simulink model "MATLABfunction"  (R2022b)
settings: Solver=FixedStepAuto  StartTime=0.0  StopTime=10.0  RelTol=1e-3
undefined symbols (not defined in the file): h, km, m, s
libraries: simulink_extras x3, aerolibconvert2 x3, autolibshared x2, vehdynlibsteering x1, simulink x1
settings Model: Creator=Lenovo  LastModifiedBy=Lenovo
settings SolverCC: EnableFixedStepZeroCrossing=on

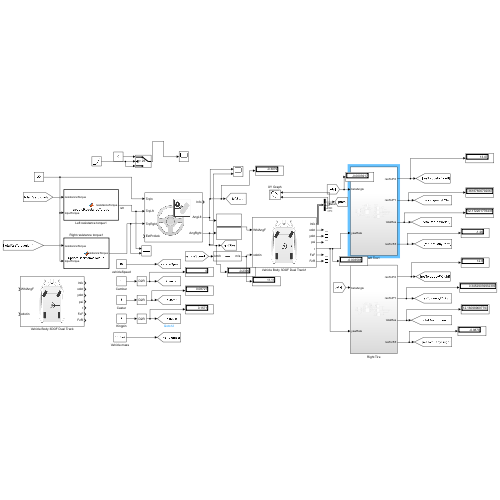
[thumbnail: Simulink's stored preview of the top-level diagram]
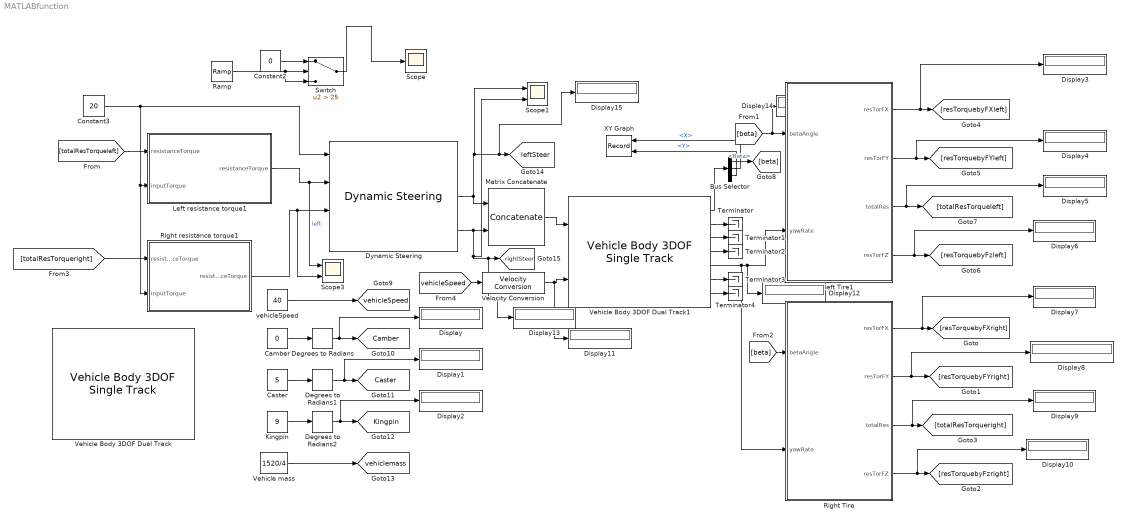
== system MATLABfunction ==
  Bus Selector : BusSelector  OutputSignals=BdyFrm.Geom.Ang.Beta,InertFrm.Cg.Disp.X,InertFrm.Cg.Disp.Y
  Camber : Constant  Value=0
  Caster : Constant  Value=5
  Constant2 : Constant  Value=0
  Constant3 : Constant  Value=20
  Degrees to Radians : simulink_extras/Transformations/Degrees to Radians
  Degrees to Radians1 : simulink_extras/Transformations/Degrees to Radians
  Degrees to Radians2 : simulink_extras/Transformations/Degrees to Radians
  Display{,1..15} (16 alike) : Display
  Dynamic Steering : vehdynlibsteering/Dynamic Steering  StrgType=Rack and pinion  StrgRatioType=Constant  PwrAst=off  Loc=Front  TrckWdth=1  WhlBase=1.524  StrgRng=1.25*pi  StrgAngBpts="[-6.2832   -5.0265   -3.7699   -2.5133   -1.2566         0    1.2566    2.5133    3.7699    5.0265    6.2832]"  StrgRatioTbl=|  StrgRatio=13.5  StrgArmLngth=0.1  RckCsLngth=0.5  TieRodLngth=0.248  D=0.2  PnnRadiusTbl="[0.0055    0.0055    0.0056    0.0057    0.0057    0.0057    0.0058    0.0057    0.0056    0.0055    0.0055]"  PnnRadius=0.0057  RodLngth=0.1  ParaArmLngth=0.9  J1=0.1  J2=0.01  beta_u=0.1  beta_l=0.1  b1=0.001  k1=30  b2=1  b3=0.001  theta_o=0  omega_o=0  FricTrq=0  TrqBpts=[-100 0 100]  VehSpdBpts=[0 20]  TrqTbl=[0 -100;0 0;0 100]  TrqLmt=100  PwrLmt=1000  Eta=1  omega_c=200  aMode=2
      | [13.5000   13.3750   13.2500   13.1250   13.0000   13.0000   13.0000   13.1250   13.2500   13.3750   13.5000
      | ]
  Kingpin : Constant  Value=9
  Left resistance torque1 : MATLAB Function  TreatAsAtomicUnit=on
  Matrix Concatenate : Concatenate  ConcatenateDimension=2
  Ramp : simulink/Sources/Ramp  slope=1  start=0  InitialOutput=5
  Right Tire : Subsystem
  Right resistance torque1 : MATLAB Function  TreatAsAtomicUnit=on
  Scope : Scope
  Scope1 : Scope  NumInputPorts=2
  Scope3 : Scope  NumInputPorts=2
  Switch : Switch  Criteria=u2 > Threshold  Threshold=25  SaturateOnIntegerOverflow=off  InputSameDT=off
  Terminator{,1..4} (5 alike) : Terminator
  Vehicle Body 3DOF Dual Track : autolibshared/Vehicle Body 3DOF Single Track  trackMode=Dual  inputMode=External longitudinal velocity  frontSteerMode=on  rearSteerMode=off  windMode=off  muMode=off  extFMode=off  extMMode=off  htchFMode=off  htchMMode=off  extXo=off  extpsio=off  extxdoto=off  extro=off  extYo=off  extTamb=off  extydoto=off  aMode=2  NF=2  NR=2  m=1520  a=1.4  b=1.6  h=0.35  dh=1  hh=0.2  X_o=0  xdot_o=0  CalphaMode=off  sigmaMode=on  d=0  hl=0  w=[1.4,1.4]  Cy_f=12e3  Cy_r=11e3  sigma_f=.1  sigma_r=.1  alpha_f_brk=[-.1 .1]  Cy_f_data=[-9e3 9e3]  alpha_r_brk=[-.1 .1]  Cy_r_data=[-9e3 9e3]  Y_o=0  ydot_o=0  Izz=4000  psi_o=0  r_o=0  Af=2  Cd=.3  Cl=.1  Cpm=.1  beta_w=[0 0.01:0.01:0.3]  Cs=[0:0.03:0.9]  Cym=[0 1e-6:0.01:0.3]  Pabs=101325  Tair=273  g=9.81  mu=1  xdot_tol=.01  Fznom=5000  Fxtire_sat=7e4  Fytire_sat=7e4  longOff=0  latOff=0  vertOff=0  wrapAng=off
      settings: LibrarySourceBlock=vehdynlibeom/Vehicle Body 3DOF Dual Track
  Vehicle Body 3DOF Dual Track1 : autolibshared/Vehicle Body 3DOF Single Track  trackMode=Dual  inputMode=External longitudinal velocity  frontSteerMode=on  rearSteerMode=off  windMode=off  muMode=off  extFMode=off  extMMode=off  htchFMode=off  htchMMode=off  extXo=off  extpsio=off  extxdoto=off  extro=off  extYo=off  extTamb=off  extydoto=off  aMode=2  NF=2  NR=2  m=1520  a=1.148  b=1.402  h=0.35  dh=1  hh=0.2  X_o=0  xdot_o=0  CalphaMode=off  sigmaMode=on  d=0  hl=0  w=[1.2,1.2]  Cy_f=350  Cy_r=12e3  sigma_f=.1  sigma_r=.1  alpha_f_brk=[-.1 .1]  Cy_f_data=[-9e3 9e3]  alpha_r_brk=[-.1 .1]  Cy_r_data=[-9e3 9e3]  Y_o=0  ydot_o=0  Izz=4000  psi_o=0  r_o=0  Af=2  Cd=.3  Cl=.1  Cpm=.1  beta_w=[0:0.01:0.3]  Cs=[0:0.03:0.9]  Cym=[0:0.01:0.3]  Pabs=101325  Tair=273  g=9.81  mu=1  xdot_tol=.01  Fznom=5000  Fxtire_sat=7e4  Fytire_sat=7e4  longOff=0  latOff=0  vertOff=0  wrapAng=off
  Vehicle mass : Constant  Value=1520/4
  Velocity Conversion : aerolibconvert2/Velocity Conversion  IU=km/h  OU=m/s
  XY Graph : Record  FileSettingsInternal="{\"entries\":[{\"content\":{\"excelSettings\":{\"content\":{},\"type\":\"Streamout.ExcelSettings\"}},\"type\":\"Streamout.FileSettingStorage\",\"uuid\":\"bec896f1-d56a-48de-90cf-f78405374d8f\"}],\"packageUris\":[\"http://schema.mathworks.com/mf0/streamout_blocks/R2020a\"],\"version\":\"1.0\"}"  Layout=[1 1]  SignalsInternal="{\"entries\":[{\"content\":{\"signals\":[{\"content\":{\"blockPath\":[\"untitled/XY Graph\"],\"channel\":[],\"dimensions\":[1],\"domain\":\"untitled/XY Graph\",\"lineColor\":\"#a2142f\",\"plots\":[1],\"port\":1,\"sid\":[\"\"],\"signalID\":30127,\"signalName\":\"<X>\"},\"type\":\"RecordBlkView.Signal\",\"uuid\":\"c8050bcf-ab5d-494c-af83-4e53599decc2\"},{\"content\":{\"blockPath\":[\"untitled/XY Graph\"],\"channel\":[],\"dimensions\":[1],\"domain\":\"untitled/XY Graph\",\"lineColor\":\"#139fff\",\"plots\":[1],\"port\":2,\"sid\":[\"\"],\"signalID\":30131,\"signalName\":\"<Y>\"},\"type\":\"RecordBlkView.Signal\",\"uuid\":\"10e66e42-d777-49f9-8d8c-30872f4fdeb7\"}]},\"type\":\"RecordBlkView.InputSignals\",\"uuid\":\"4fc47762-2255-40e3-9f9f-7b4ae2eb3bc2\"}],\"packageUris\":[\"http://schema.mathworks.com/mf0/streamout_blocks/R2020a\"],\"version\":\"1.0\"}"  VisualizationBindings="{\"xyplotplugin\":{\"info\":[{\"series\":[{\"bindingParametersList\":[{\"parameter\":\"X-Axis\",\"signalID\":30127,\"signalName\":\"<X>\"},{\"parameter\":\"Y-Axis\",\"signalID\":30131,\"signalName\":\"<Y>\"}],\"seriesID\":15033}],\"subplotID\":1}]}}"  CompatibilityTag=XY
  left Tire1 : Subsystem
  vehicleSpeed : Constant  Value=40
  tag scope: Camber=global, Caster=global, Kingpin=global, leftSteer=global, rightSteer=global, vehicleSpeed=global, vehiclemass=global
  wires:
  [beta] -> Right Tire/1(betaAngle)
  Dynamic Steering/2 -> Matrix Concatenate/1, Scope1/1, Display15/1, [leftSteer]
  Dynamic Steering/3 -> Scope1/2, [rightSteer], Display13/1, Matrix Concatenate/2
  Matrix Concatenate/1 -> Vehicle Body 3DOF Dual Track1/1
  Right Tire/1(resTorFX) -> Display7/1, [resTorquebyFXright]
  Right Tire/2(resTorFY) -> Display8/1, [resTorquebyFYright]
  Right Tire/4(resTorFZ) -> Display10/1, [resTorquebyFzright]
  Right Tire/3(totalRes) -> Display9/1, [totalResTorqueright]
  Vehicle Body 3DOF Dual Track1/5 -> Display12/1, left Tire1/2(yawRate), Right Tire/2(yawRate)
  Vehicle Body 3DOF Dual Track1/1 -> Bus Selector/1
  Bus Selector/1 -> [beta]  "<Beta>"
  [beta] -> Display14/1, left Tire1/1(betaAngle)
  Vehicle Body 3DOF Dual Track1/2 -> Terminator/1
  Vehicle Body 3DOF Dual Track1/3 -> Terminator1/1
  Vehicle Body 3DOF Dual Track1/4 -> Terminator2/1
  Vehicle Body 3DOF Dual Track1/6 -> Terminator3/1
  Vehicle Body 3DOF Dual Track1/7 -> Terminator4/1
  vehicleSpeed/1 -> [vehicleSpeed]
  Camber/1 -> Degrees to Radians/1
  Caster/1 -> Degrees to Radians1/1
  Kingpin/1 -> Degrees to Radians2/1
  Vehicle mass/1 -> [vehiclemass]
  Degrees to Radians/1 -> Display/1, [Camber]
  Degrees to Radians1/1 -> Display1/1, [Caster]
  Degrees to Radians2/1 -> Display2/1, [Kingpin]
  [vehicleSpeed] -> Velocity Conversion/1
  Velocity Conversion/1 -> Display11/1, Vehicle Body 3DOF Dual Track1/2
  Constant2/1 -> Switch/1
  Ramp/1 -> Switch/3, Switch/2
  Switch/1 -> Scope/1
  Bus Selector/2 -> XY Graph/1  "<X>"
  Bus Selector/3 -> XY Graph/2  "<Y>"
  left Tire1/3(totalRes) -> Display5/1, [totalResTorqueleft]
  left Tire1/4(resTorFZ) -> Display6/1, [resTorquebyFzleft]
  left Tire1/2(resTorFY) -> Display4/1, [resTorquebyFYleft]
  left Tire1/1(resTorFX) -> Display3/1, [resTorquebyFXleft]
  [totalResTorqueleft] -> Left resistance torque1/1("resistanceTorque ")
  Constant3/1 -> Right resistance torque1/2(inputTorque), Left resistance torque1/2(inputTorque), Dynamic Steering/1
  Left resistance torque1/1(resistanceTorque) -> Scope3/1, Dynamic Steering/2  "left"
  [totalResTorqueright] -> Right resistance torque1/1("resistanceTorque ")
  Right resistance torque1/1(resistanceTorque) -> Scope3/2, Dynamic Steering/3

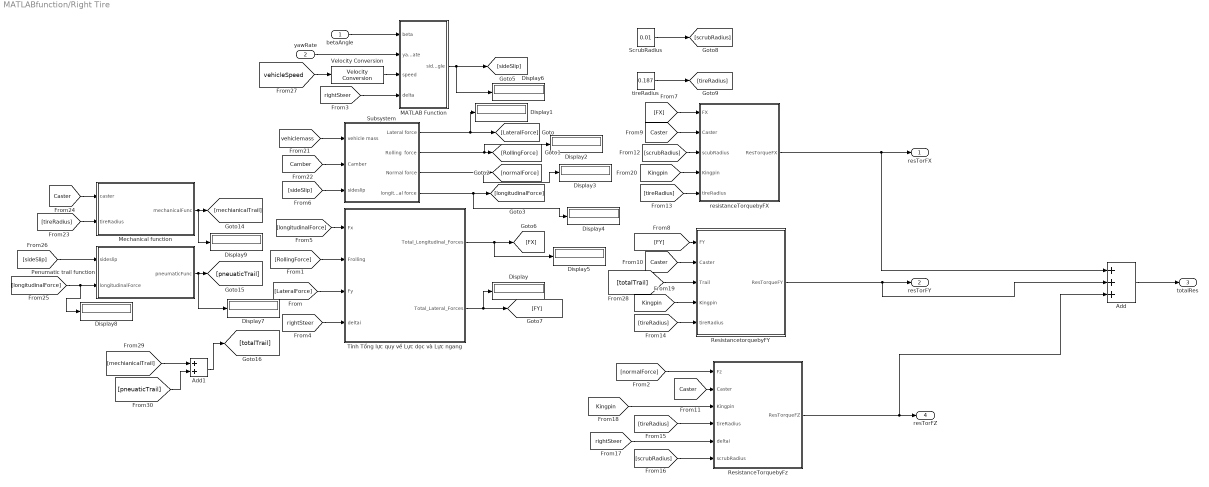
== system MATLABfunction/Right Tire ==
  betaAngle : Inport
  yawRate : Inport  Port=2
  Add : Sum  Inputs=+++
  Add1 : Sum
  Display{,1..9} (10 alike) : Display
  MATLAB Function : MATLAB Function  TreatAsAtomicUnit=on
  Mechanical function : MATLAB Function  TreatAsAtomicUnit=on
  Penumatic trail function : MATLAB Function  TreatAsAtomicUnit=on
  ResistanceTorquebyFz : MATLAB Function  TreatAsAtomicUnit=on
  ResistancetorquebyFY : MATLAB Function  TreatAsAtomicUnit=on
  ScrubRadius : Constant  Value=0.01
  Subsystem : Subsystem
  Tính Tổng lực quy về Lực dọc và Lực ngang : Subsystem
  Velocity Conversion : aerolibconvert2/Velocity Conversion  IU=km/h  OU=m/s
  resistanceTorquebyFX : MATLAB Function  TreatAsAtomicUnit=on
  tireRadius : Constant  Value=0.187
  resTorFX : Outport
  resTorFY : Outport  Port=2
  totalRes : Outport  Port=3
  resTorFZ : Outport  Port=4
  wires:
  [longitudinalForce] -> Display8/1, Penumatic trail function/2(longitudinalForce)
  [Camber] -> Subsystem/2(Camber)
  [tireRadius] -> resistanceTorquebyFX/5(tireRadius)
  tireRadius/1 -> [tireRadius]
  [normalForce] -> ResistanceTorquebyFz/1(Fz)
  Subsystem/4(longitudinal force) -> Display4/1, [longitudinalForce]
  [Caster] -> ResistanceTorquebyFz/2(Caster)
  [RollingForce] -> Tính Tổng lực quy về Lực dọc và Lực ngang/2(Frolling)
  Subsystem/3(Normal force) -> Display3/1, [normalForce]
  [Caster] -> resistanceTorquebyFX/2(Caster)
  resistanceTorquebyFX/1(ResTorqueFX) -> resTorFX/1, Add/1
  [scrubRadius] -> resistanceTorquebyFX/3(scubRadius)
  Subsystem/1(Lateral force) -> Display1/1, [LateralForce]
  Tính Tổng lực quy về Lực dọc và Lực ngang/1(Total_Longitudinal_Forces) -> Display5/1, [FX]
  MATLAB Function/1(sideslipAngle) -> Display6/1, [sideSlip]
  Mechanical function/1(mechanicalFunc) -> Display9/1, [mechianicalTrail]
  [sideSlip] -> Subsystem/3(sideslip)
  [Kingpin] -> ResistancetorquebyFY/4(Kingpin)
  [Kingpin] -> resistanceTorquebyFX/4(Kingpin)
  ResistanceTorquebyFz/1(ResTorqueFZ) -> resTorFZ/1, Add/3
  Add/1 -> totalRes/1
  [totalTrail] -> ResistancetorquebyFY/3(Trail)
  [longitudinalForce] -> Tính Tổng lực quy về Lực dọc và Lực ngang/1(Fx)
  [tireRadius] -> Mechanical function/2(tireRadius)
  ResistancetorquebyFY/1(ResTorqueFY) -> resTorFY/1, Add/2
  [scrubRadius] -> ResistanceTorquebyFz/6(scrubRadius)
  [vehiclemass] -> Subsystem/1(vehicle mass)
  Tính Tổng lực quy về Lực dọc và Lực ngang/2(Total_Lateral_Forces) -> Display/1, [FY]
  Subsystem/2(Rolling  force) -> Display2/1, [RollingForce]
  [rightSteer] -> MATLAB Function/4(delta)
  [rightSteer] -> Tính Tổng lực quy về Lực dọc và Lực ngang/4(deltai)
  Penumatic trail function/1(pneumaticFunc) -> Display7/1, [pneuaticTrail]
  [LateralForce] -> Tính Tổng lực quy về Lực dọc và Lực ngang/3(Fy)
  [rightSteer] -> ResistanceTorquebyFz/5(deltai)
  [sideSlip] -> Penumatic trail function/1(sideslip)
  ScrubRadius/1 -> [scrubRadius]
  [tireRadius] -> ResistancetorquebyFY/5(tireRadius)
  [FX] -> resistanceTorquebyFX/1(FX)
  [Caster] -> ResistancetorquebyFY/2(Caster)
  [tireRadius] -> ResistanceTorquebyFz/4(tireRadius)
  [FY] -> ResistancetorquebyFY/1(FY)
  [vehicleSpeed] -> Velocity Conversion/1
  [Kingpin] -> ResistanceTorquebyFz/3(Kingpin)
  betaAngle/1 -> MATLAB Function/1(beta)
  [Caster] -> Mechanical function/1(caster)
  yawRate/1 -> MATLAB Function/2(yawRate)
  Velocity Conversion/1 -> MATLAB Function/3(speed)
  [mechianicalTrail] -> Add1/1
  Add1/1 -> [totalTrail]
  [pneuaticTrail] -> Add1/2

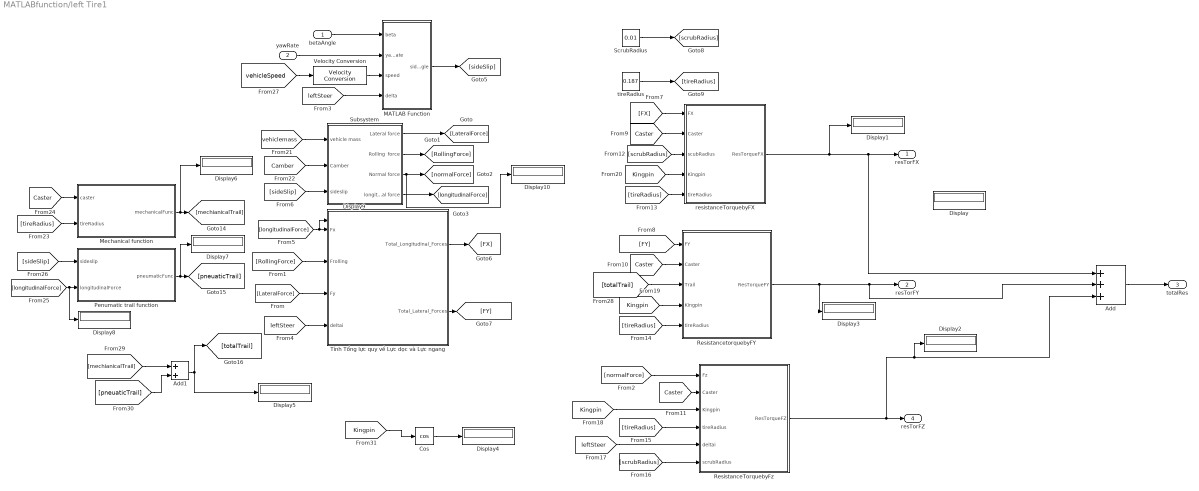
== system MATLABfunction/left Tire1 ==
  betaAngle : Inport
  yawRate : Inport  Port=2
  Add : Sum  Inputs=+++
  Add1 : Sum
  Cos : Trigonometry  Operator=cos
  Display{,1..10} (11 alike) : Display
  MATLAB Function : MATLAB Function  TreatAsAtomicUnit=on
  Mechanical function : MATLAB Function  TreatAsAtomicUnit=on
  Penumatic trail function : MATLAB Function  TreatAsAtomicUnit=on
  ResistanceTorquebyFz : MATLAB Function  TreatAsAtomicUnit=on
  ResistancetorquebyFY : MATLAB Function  TreatAsAtomicUnit=on
  ScrubRadius : Constant  Value=0.01
  Subsystem : Subsystem
  Tính Tổng lực quy về Lực dọc và Lực ngang : Subsystem
  Velocity Conversion : aerolibconvert2/Velocity Conversion  IU=km/h  OU=m/s
  resistanceTorquebyFX : MATLAB Function  TreatAsAtomicUnit=on
  tireRadius : Constant  Value=0.187
  resTorFX : Outport
  resTorFY : Outport  Port=2
  totalRes : Outport  Port=3
  resTorFZ : Outport  Port=4
  wires:
  [pneuaticTrail] -> Add1/2
  Add1/1 -> [totalTrail], Display5/1
  [mechianicalTrail] -> Add1/1
  Velocity Conversion/1 -> MATLAB Function/3(speed)
  yawRate/1 -> MATLAB Function/2(yawRate)
  [Caster] -> Mechanical function/1(caster)
  betaAngle/1 -> MATLAB Function/1(beta)
  [Kingpin] -> ResistanceTorquebyFz/3(Kingpin)
  [vehicleSpeed] -> Velocity Conversion/1
  [FY] -> ResistancetorquebyFY/1(FY)
  [tireRadius] -> ResistanceTorquebyFz/4(tireRadius)
  [Caster] -> ResistancetorquebyFY/2(Caster)
  [FX] -> resistanceTorquebyFX/1(FX)
  [tireRadius] -> ResistancetorquebyFY/5(tireRadius)
  ScrubRadius/1 -> [scrubRadius]
  [sideSlip] -> Penumatic trail function/1(sideslip)
  [leftSteer] -> ResistanceTorquebyFz/5(deltai)
  [LateralForce] -> Tính Tổng lực quy về Lực dọc và Lực ngang/3(Fy)
  Penumatic trail function/1(pneumaticFunc) -> Display7/1, [pneuaticTrail]
  [leftSteer] -> Tính Tổng lực quy về Lực dọc và Lực ngang/4(deltai)
  [leftSteer] -> MATLAB Function/4(delta)
  Subsystem/2(Rolling  force) -> [RollingForce]
  Tính Tổng lực quy về Lực dọc và Lực ngang/2(Total_Lateral_Forces) -> [FY]
  [vehiclemass] -> Subsystem/1(vehicle mass)
  [scrubRadius] -> ResistanceTorquebyFz/6(scrubRadius)
  ResistancetorquebyFY/1(ResTorqueFY) -> Display3/1, Add/2, resTorFY/1
  [tireRadius] -> Mechanical function/2(tireRadius)
  [longitudinalForce] -> Display9/1, Tính Tổng lực quy về Lực dọc và Lực ngang/1(Fx)
  [totalTrail] -> ResistancetorquebyFY/3(Trail)
  Add/1 -> totalRes/1
  ResistanceTorquebyFz/1(ResTorqueFZ) -> Display2/1, Add/3, resTorFZ/1
  [Kingpin] -> resistanceTorquebyFX/4(Kingpin)
  [Kingpin] -> ResistancetorquebyFY/4(Kingpin)
  [sideSlip] -> Subsystem/3(sideslip)
  Mechanical function/1(mechanicalFunc) -> Display6/1, [mechianicalTrail]
  MATLAB Function/1(sideslipAngle) -> [sideSlip]
  Tính Tổng lực quy về Lực dọc và Lực ngang/1(Total_Longitudinal_Forces) -> [FX]
  Subsystem/1(Lateral force) -> [LateralForce]
  [scrubRadius] -> resistanceTorquebyFX/3(scubRadius)
  resistanceTorquebyFX/1(ResTorqueFX) -> Display1/1, Add/1, resTorFX/1
  [Caster] -> resistanceTorquebyFX/2(Caster)
  Subsystem/3(Normal force) -> Display10/1, [normalForce]
  [RollingForce] -> Tính Tổng lực quy về Lực dọc và Lực ngang/2(Frolling)
  [Caster] -> ResistanceTorquebyFz/2(Caster)
  Subsystem/4(longitudinal force) -> [longitudinalForce]
  [normalForce] -> ResistanceTorquebyFz/1(Fz)
  tireRadius/1 -> [tireRadius]
  [tireRadius] -> resistanceTorquebyFX/5(tireRadius)
  [Camber] -> Subsystem/2(Camber)
  [longitudinalForce] -> Display8/1, Penumatic trail function/2(longitudinalForce)
  [Kingpin] -> Cos/1
  Cos/1 -> Display4/1

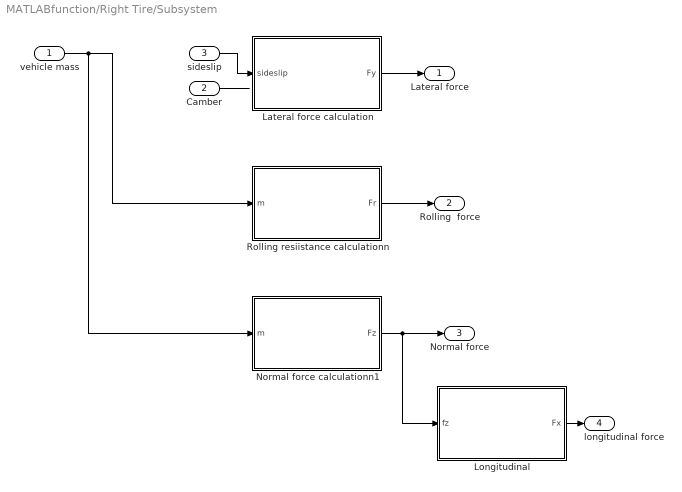
== system MATLABfunction/Right Tire/Subsystem ==
  vehicle mass : Inport
  Camber : Inport  Port=2
  sideslip : Inport  Port=3
  Lateral force calculation : MATLAB Function  TreatAsAtomicUnit=on
  Longitudinal : MATLAB Function  TreatAsAtomicUnit=on
  Normal force calculationn1 : MATLAB Function  TreatAsAtomicUnit=on
  Rolling resiistance calculationn : MATLAB Function  TreatAsAtomicUnit=on
  Lateral force : Outport
  Rolling  force : Outport  Port=2
  Normal force : Outport  Port=3
  longitudinal force : Outport  Port=4
  wires:
  Lateral force calculation/1(Fy) -> Lateral force/1
  vehicle mass/1 -> Normal force calculationn1/1(m), Rolling resiistance calculationn/1(m)
  Normal force calculationn1/1(Fz) -> Normal force/1, Longitudinal/1(fz)
  Rolling resiistance calculationn/1(Fr) -> Rolling  force/1
  Camber/1 -> ?
  Longitudinal/1(Fx) -> longitudinal force/1
  sideslip/1 -> Lateral force calculation/1(sideslip)

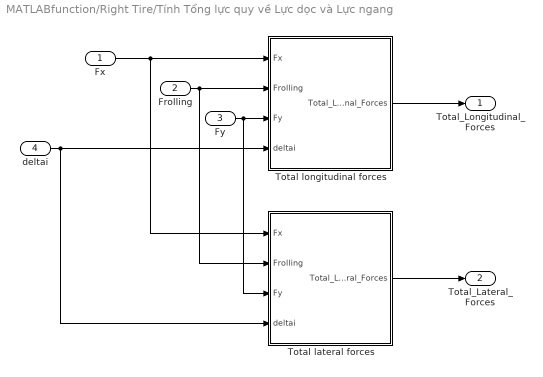
== system MATLABfunction/Right Tire/Tính Tổng lực quy về Lực dọc và Lực ngang ==
  Fx : Inport
  Frolling : Inport  Port=2
  Fy : Inport  Port=3
  deltai : Inport  Port=4
  Total lateral forces : MATLAB Function  TreatAsAtomicUnit=on
  Total longitudinal forces : MATLAB Function  TreatAsAtomicUnit=on
  Total_Longitudinal_Forces : Outport
  Total_Lateral_Forces : Outport  Port=2
  wires:
  deltai/1 -> Total lateral forces/4(deltai), Total longitudinal forces/4(deltai)
  Fy/1 -> Total lateral forces/3(Fy), Total longitudinal forces/3(Fy)
  Frolling/1 -> Total lateral forces/2(Frolling), Total longitudinal forces/2(Frolling)
  Total lateral forces/1(Total_Lateral_Forces) -> Total_Lateral_Forces/1
  Fx/1 -> Total longitudinal forces/1(Fx), Total lateral forces/1(Fx)
  Total longitudinal forces/1(Total_Longitudinal_Forces) -> Total_Longitudinal_Forces/1

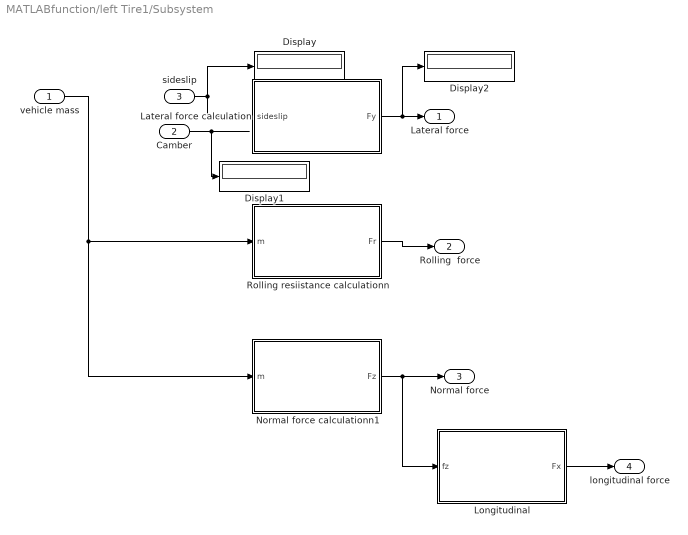
== system MATLABfunction/left Tire1/Subsystem ==
  vehicle mass : Inport
  Camber : Inport  Port=2
  sideslip : Inport  Port=3
  Display : Display
  Display1 : Display
  Display2 : Display
  Lateral force calculation : MATLAB Function  TreatAsAtomicUnit=on
  Longitudinal : MATLAB Function  TreatAsAtomicUnit=on
  Normal force calculationn1 : MATLAB Function  TreatAsAtomicUnit=on
  Rolling resiistance calculationn : MATLAB Function  TreatAsAtomicUnit=on
  Lateral force : Outport
  Rolling  force : Outport  Port=2
  Normal force : Outport  Port=3
  longitudinal force : Outport  Port=4
  wires:
  sideslip/1 -> Display/1, Lateral force calculation/1(sideslip)
  Longitudinal/1(Fx) -> longitudinal force/1
  Camber/1 -> Display1/1
  Rolling resiistance calculationn/1(Fr) -> Rolling  force/1
  Normal force calculationn1/1(Fz) -> Longitudinal/1(fz), Normal force/1
  vehicle mass/1 -> Rolling resiistance calculationn/1(m), Normal force calculationn1/1(m)
  Lateral force calculation/1(Fy) -> Display2/1, Lateral force/1

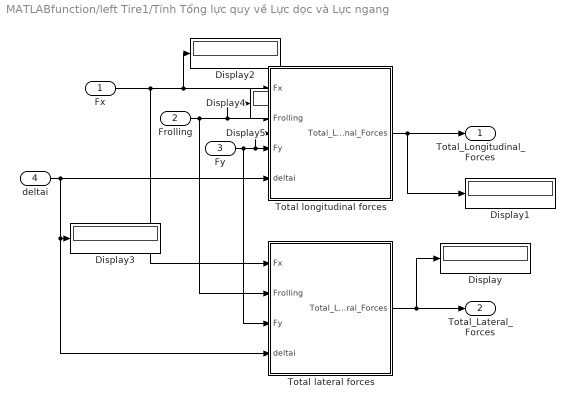
== system MATLABfunction/left Tire1/Tính Tổng lực quy về Lực dọc và Lực ngang ==
  Fx : Inport
  Frolling : Inport  Port=2
  Fy : Inport  Port=3
  deltai : Inport  Port=4
  Display{,1..5} (6 alike) : Display
  Total lateral forces : MATLAB Function  TreatAsAtomicUnit=on
  Total longitudinal forces : MATLAB Function  TreatAsAtomicUnit=on
  Total_Longitudinal_Forces : Outport
  Total_Lateral_Forces : Outport  Port=2
  wires:
  Total longitudinal forces/1(Total_Longitudinal_Forces) -> Total_Longitudinal_Forces/1, Display1/1
  Fx/1 -> Total lateral forces/1(Fx), Display2/1, Total longitudinal forces/1(Fx)
  Total lateral forces/1(Total_Lateral_Forces) -> Display/1, Total_Lateral_Forces/1
  Frolling/1 -> Display4/1, Total longitudinal forces/2(Frolling), Total lateral forces/2(Frolling)
  deltai/1 -> Total longitudinal forces/4(deltai), Display3/1, Total lateral forces/4(deltai)
  Fy/1 -> Display5/1, Total longitudinal forces/3(Fy), Total lateral forces/3(Fy)

== matlab function MATLABfunction/Right Tire/Mechanical function ==
  data: caster input; mechanicalFunc output; tireRadius input
function mechanicalFunc = fcn(caster,tireRadius)


mechanicalFunc = sin(caster) * tireRadius;

== matlab function MATLABfunction/Right Tire/Penumatic trail function ==
  data: sideslip input; pneumaticFunc output; longitudinalForce input
function pneumaticFunc = fcn(sideslip,longitudinalForce)


%khai  bao Tp0
initialTrail = 0.03;
corneringStiffness = 350;

pneumaticFunc = initialTrail * (1 - sign(sideslip)*(corneringStiffness/(3*longitudinalForce))*tan(sideslip));

== matlab function MATLABfunction/Right Tire/Subsystem/Rolling resiistance calculationn ==
  data: m input; Fr output
function Fr = fcn(m)

% Khai báo các hằng số Cα và Cγ
g = 9.81;
f = 0.011;


% Tính toán lực dọc Fy
Fr = m*g*f;

== matlab function MATLABfunction/left Tire1/MATLAB Function ==
  data: beta input; sideslipAngle output; yawRate input; speed input; delta input
function sideslipAngle = fcn(beta,yawRate,speed,delta)


%khai bao a1
a1 = 1.148;

sideslipAngle = beta + ((a1*yawRate)/speed) -delta;

== matlab function MATLABfunction/left Tire1/Mechanical function ==
  data: caster input; mechanicalFunc output; tireRadius input
function mechanicalFunc = fcn(caster,tireRadius)


mechanicalFunc = sin(caster) * tireRadius;

== matlab function MATLABfunction/left Tire1/Penumatic trail function ==
  data: sideslip input; pneumaticFunc output; longitudinalForce input
function pneumaticFunc = fcn(sideslip,longitudinalForce)


%khai  bao Tp0
initialTrail = 0.03;
corneringStiffness = 350;


pneumaticFunc = initialTrail * (1 - sign(sideslip)*(corneringStiffness/(3*longitudinalForce))*tan(sideslip));

== matlab function MATLABfunction/left Tire1/ResistanceTorquebyFz ==
  data: Fz input; ResTorqueFZ output; Caster input; Kingpin input; tireRadius input; deltai input; scrubRadius input
function ResTorqueFZ = fcn(Fz,Caster,Kingpin,tireRadius,deltai,scrubRadius)





% Tính toán lực dọc F_X
ResTorqueFZ = Fz * sin(Kingpin)*cos(Caster)*sin(deltai)*cos(Kingpin)* (tireRadius * tan(Caster) + scrubRadius);

== matlab function MATLABfunction/left Tire1/ResistancetorquebyFY ==
  data: FY input; ResTorqueFY output; Caster input; Trail input; Kingpin input; tireRadius input
function ResTorqueFY = fcn(FY,Caster,Trail,Kingpin,tireRadius)





% Tính toán lực dọc F_X
ResTorqueFY = FY * cos(Kingpin)* (Trail*cos(Caster) + tireRadius * sin(Caster));

== matlab function MATLABfunction/left Tire1/Subsystem/Lateral force calculation ==
  data: sideslip input; Fy output
function Fy = fcn(sideslip)%camber)

% Khai báo các hằng số Cα và Cγ
Ca = 350;
Cy = 140;


% Tính toán lực dọc Fy
Fy = Ca *sideslip; % Cy * camber;

== matlab function MATLABfunction/left Tire1/Subsystem/Longitudinal ==
  data: fz input; Fx output
function Fx = fcn(fz)

% Khai báo các hằng số Cα và Cγ
Us = 0.35;


% Tính toán lực dọc Fy
Fx = Us * fz;

== matlab function MATLABfunction/left Tire1/Subsystem/Normal force calculationn1 ==
  data: m input; Fz output
function Fz = fcn(m)

% Khai báo các hằng số Cα và Cγ
g = 9.81;
a2 = 1.402;
l = 2.55;


% Tính toán lực dọc Fy
Fz = (1/2)*m*g*(a2/l);

== matlab function MATLABfunction/Right Tire/Subsystem/Lateral force calculation ==
  data: sideslip input; Fy output
function Fy = fcn(sideslip)

% Khai báo các hằng số Cα và Cγ
Ca = 350;
Cy = 140;


% Tính toán lực dọc Fy
Fy = Ca *sideslip;

== matlab function MATLABfunction/left Tire1/Subsystem/Rolling resiistance calculationn ==
  data: m input; Fr output
function Fr = fcn(m)

% Khai báo các hằng số Cα và Cγ
g = 9.81;
f = 0.011;


% Tính toán lực dọc Fy
Fr = m*g*f;

== matlab function MATLABfunction/left Tire1/Tính Tổng lực quy về Lực dọc và Lực ngang/Total lateral forces ==
  data: Fx input; Total_Lateral_Forces output; Frolling input; Fy input; deltai input
function Total_Lateral_Forces = fcn(Fx,Frolling,Fy,deltai)





% Tính toán lực dọc F_X
Total_Lateral_Forces = Fy*cos(deltai) + (Fx - Frolling)*sin(deltai);

== matlab function MATLABfunction/left Tire1/Tính Tổng lực quy về Lực dọc và Lực ngang/Total longitudinal forces ==
  data: Fx input; Total_Longitudinal_Forces output; Frolling input; Fy input; deltai input
function Total_Longitudinal_Forces = fcn(Fx,Frolling,Fy,deltai)


% Tính toán lực dọc F_X
Total_Longitudinal_Forces = (Fx - Frolling) * cos(deltai) - Fy * sin(deltai);

== matlab function MATLABfunction/left Tire1/resistanceTorquebyFX ==
  data: FX input; ResTorqueFX output; Caster input; scubRadius input; Kingpin input; tireRadius input
function ResTorqueFX = fcn(FX,Caster,scubRadius,Kingpin,tireRadius)





% Tính toán lực dọc F_X
ResTorqueFX = FX * cos(Caster)* (scubRadius*cos(Kingpin) + tireRadius * sin(Kingpin));

== matlab function MATLABfunction/Left resistance torque1 ==
  data: resistanceTorque input; resistanceTorque output; inputTorque input
function resistanceTorque = updateResistanceTorque(resistanceTorque, inputTorque)
    if inputTorque >= 0
        resistanceTorque = resistanceTorque * -1;
    else
        resistanceTorque = resistanceTorque;
    end
end

== matlab function MATLABfunction/Right resistance torque1 ==
  data: resistanceTorque input; resistanceTorque output; inputTorque input
function resistanceTorque = updateResistanceTorque(resistanceTorque, inputTorque)
    if inputTorque > 0
        resistanceTorque = resistanceTorque * -1;
    else
        resistanceTorque = resistanceTorque;
    end
end

== matlab function MATLABfunction/Right Tire/Subsystem/Normal force calculationn1 ==
  data: m input; Fz output
function Fz = fcn(m)

% Khai báo các hằng số Cα và Cγ
g = 9.81;
a2 = 1.402;
l = 2.55;


% Tính toán lực dọc Fy
Fz = (1/2)*m*g*(a2/l);

== matlab function MATLABfunction/Right Tire/Subsystem/Longitudinal ==
  data: fz input; Fx output
function Fx = fcn(fz)

% Khai báo các hằng số Cα và Cγ
Us = 0.35;


% Tính toán lực dọc Fy
Fx = Us * fz;

== matlab function MATLABfunction/Right Tire/Tính Tổng lực quy về Lực dọc và Lực ngang/Total longitudinal forces ==
  data: Fx input; Total_Longitudinal_Forces output; Frolling input; Fy input; deltai input
function Total_Longitudinal_Forces = fcn(Fx,Frolling,Fy,deltai)





% Tính toán lực dọc F_X
Total_Longitudinal_Forces = (Fx - Frolling) * cos(deltai) - Fy * sin(deltai);

== matlab function MATLABfunction/Right Tire/Tính Tổng lực quy về Lực dọc và Lực ngang/Total lateral forces ==
  data: Fx input; Total_Lateral_Forces output; Frolling input; Fy input; deltai input
function Total_Lateral_Forces = fcn(Fx,Frolling,Fy,deltai)





% Tính toán lực dọc F_X
Total_Lateral_Forces = Fy*cos(deltai) + (Fx - Frolling)*sin(deltai);

== matlab function MATLABfunction/Right Tire/resistanceTorquebyFX ==
  data: FX input; ResTorqueFX output; Caster input; scubRadius input; Kingpin input; tireRadius input
function ResTorqueFX = fcn(FX,Caster,scubRadius,Kingpin,tireRadius)





% Tính toán lực dọc F_X
ResTorqueFX = FX * cos(Caster)* (scubRadius*cos(Kingpin) + tireRadius * sin(Kingpin));

== matlab function MATLABfunction/Right Tire/ResistancetorquebyFY ==
  data: FY input; ResTorqueFY output; Caster input; Trail input; Kingpin input; tireRadius input
function ResTorqueFY = fcn(FY,Caster,Trail,Kingpin,tireRadius)





% Tính toán lực dọc F_X
ResTorqueFY = FY * cos(Kingpin)* (Trail*cos(Caster) + tireRadius * sin(Caster));

== matlab function MATLABfunction/Right Tire/ResistanceTorquebyFz ==
  data: Fz input; ResTorqueFZ output; Caster input; Kingpin input; tireRadius input; deltai input; scrubRadius input
function ResTorqueFZ = fcn(Fz,Caster,Kingpin,tireRadius,deltai,scrubRadius)





% Tính toán lực dọc F_X
ResTorqueFZ = Fz * sin(Kingpin)*cos(Caster)*sin(deltai)*cos(Kingpin)* (tireRadius * tan(Caster) + scrubRadius);

== matlab function MATLABfunction/Right Tire/MATLAB Function ==
  data: beta input; sideslipAngle output; yawRate input; speed input; delta input
function sideslipAngle = fcn(beta,yawRate,speed,delta)


%khai bao a1
a1 = 1.148;

sideslipAngle = beta + ((a1*yawRate)/speed) -delta;
